simulink model "DK_sim_LFR_diferencial"  (R2020b)
settings: Solver=VariableStepAuto  StartTime=0.0  StopTime=inf  RelTol=1e-3
libraries: vrlib x3
settings Model: Creator=ponyj  LastModifiedBy=ponyj

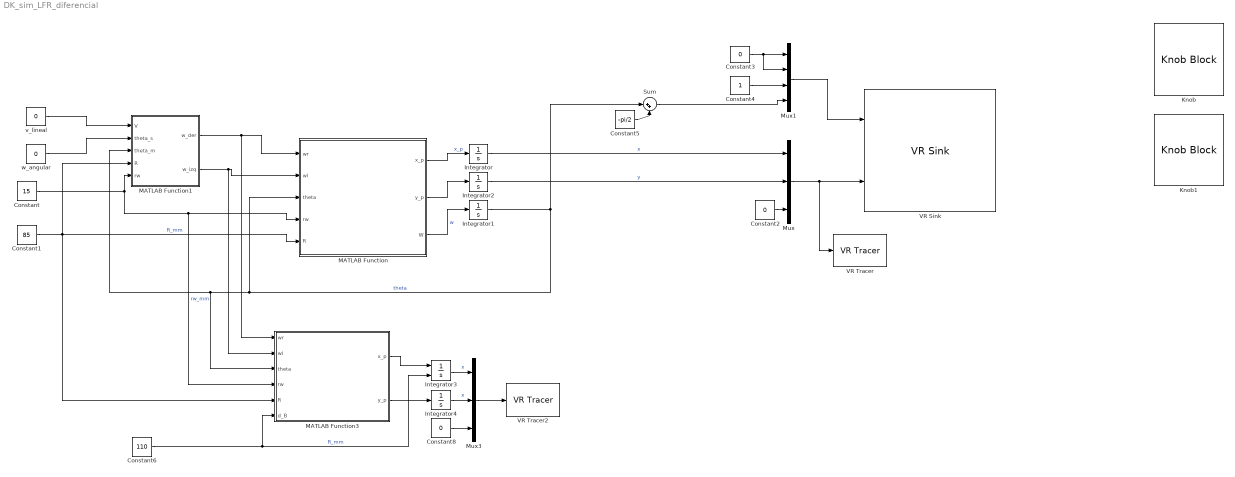
== system DK_sim_LFR_diferencial ==
  Constant : Constant  Value=15
  Constant1 : Constant  Value=85
  Constant2 : Constant  Value=0
  Constant3 : Constant  Value=0
  Constant4 : Constant
  Constant5 : Constant  Value=-pi/2
  Constant6 : Constant  Value=110
  Constant8 : Constant  Value=0
  Integrator{,1..2,4} (4 alike) : Integrator
  Integrator3 : Integrator  InitialConditionSource=external  InitialCondition=1
  Knob : KnobBlock  ScaleMin=-50  ScaleMax=50
  Knob1 : KnobBlock  ScaleMin=-360  ScaleMax=360
  MATLAB Function : MATLAB Function  TreatAsAtomicUnit=on
  MATLAB Function1 : MATLAB Function  TreatAsAtomicUnit=on
  MATLAB Function3 : MATLAB Function  TreatAsAtomicUnit=on
  Mux : Mux  Inputs=3
  Mux1 : Mux
  Mux3 : Mux  Inputs=3
  Sum : Sum  Inputs=|++
  VR Sink : vrlib/VR Sink  InstantiateOnLoad=on  SampleTime=0.1  ViewEnable=on  RemoteChange=off  RemoteView=off  FieldsWritten=LFR_carro.rotation.4.1.1.double#LFR_carro.translation.3.1.1.double  WorldFileName=Mod_Seg_config.wrl  AutoView=off  VideoDimensions=[]  AllowVariableSize=off  FigureProperties="{'Position', 'Name', 'Viewpoint', 'CameraBound', 'CameraDirection', 'CameraPosition', 'CameraUpVector', 'ZoomFactor', 'Antialiasing', 'Headlight', 'Lighting', 'NavPanel', 'Sound', 'StatusBar', 'Stereo3D', 'Stereo3DCameraOffset', 'Stereo3DHIT', 'ToolBar', 'Textures', 'Transparency', 'Triad', 'Wireframe', 'NavZones', 'NavMode', 'NavSpeed', 'CaptureFileFormat', 'CaptureFileName', 'Record2DCompressMethod', 'Record2DCompressQuality', 'Record2D', 'Record2DFileName', 'Record2DFPS'; [1.8000000000000000e+00   8.1399999999999977e+01   7.6640000000000009e+02   6.8280000000000007e+02], '', '_untitled_1', 'on', [0.0000000000000000e+00   0.0000000000000000e+00  -1.0000000000000000e+00], [0.0000000000000000e+00   0.0000000000000000e+00   0.0000000000000000e+00], [0.0000000000000000e+00   1.0000000000000000e+00   0.0000000000000000e+00], [1.0000000000000000e+00], 'on', 'on', 'on', 'halfbar', 'on', 'on', 'off', [1.0000000149011612e-01], [0.0000000000000000e+00], 'on', 'on', 'on', 'none', 'off', 'off', 'fly', 'normal', 'tif', '%f_anim_%n.tif', 'auto', [7.5000000000000000e+01], 'off', '%f_anim_%n.avi', 'auto'}"
  VR Tracer : vrlib/VR Tracer  VrmlFile=Mod_Seg_config.wrl  MarkerName=Tetrahedron  UseLines=on  UseTriads=on  MarkerScale=[1 1 1]  MarkerColorSelection=Selected from color list  MarkerColor=green  rgbval=[1 0 0]  Ts=0.5  ForceViewerOpen=off  ConnectPlane=off  PlaneCoeff=[0 1 0 0]  ConnectPoint=None  PointCoord=[0 0 0]
      settings: SourceProductBaseCode=SL
  VR Tracer2 : vrlib/VR Tracer  VrmlFile=Mod_Seg_config.wrl  MarkerName=Tetrahedron  UseLines=on  UseTriads=on  MarkerScale=[1 1 1]  MarkerColorSelection=Selected from color list  MarkerColor=yellow  rgbval=[1 0 0]  Ts=0.5  ForceViewerOpen=off  ConnectPlane=off  PlaneCoeff=[0 1 0 0]  ConnectPoint=None  PointCoord=[0 0 0]
      settings: SourceProductBaseCode=SL
  v_lineal : Constant  Value=0
  w_angular : Constant  Value=0
  wires:
  Constant/1 -> MATLAB Function3/4(rw), MATLAB Function/4(rw), MATLAB Function1/5(rw)  "rw_mm"
  Constant1/1 -> MATLAB Function3/5(R), MATLAB Function/5(R), MATLAB Function1/4(R)  "R_mm"
  MATLAB Function/1(x_p) -> Integrator/1  "x_p"
  MATLAB Function/3(W) -> Integrator1/1  "w"
  Integrator/1 -> Mux/1  "x"
  Integrator1/1 -> MATLAB Function/3(theta), MATLAB Function3/3(theta), MATLAB Function1/3(theta_m), Sum/1  "theta"
  Mux/1 -> VR Tracer/1, VR Sink/2
  Integrator2/1 -> Mux/2  "y"
  Constant2/1 -> Mux/3
  Mux1/1 -> VR Sink/1
  Constant4/1 -> Mux1/3
  Constant3/1 -> Mux1/2, Mux1/1
  Sum/1 -> Mux1/4
  Constant5/1 -> Sum/2
  v_lineal/1 -> MATLAB Function1/1(V)
  w_angular/1 -> MATLAB Function1/2(theta_s)
  MATLAB Function1/1(w_der) -> MATLAB Function3/1(wr), MATLAB Function/1(wr)
  MATLAB Function/2(y_p) -> Integrator2/1
  Constant6/1 -> Integrator3/2, MATLAB Function3/6(d_B)  "R_mm"
  MATLAB Function1/2(w_izq) -> MATLAB Function/2(wl), MATLAB Function3/2(wl)
  Mux3/1 -> VR Tracer2/1
  Constant8/1 -> Mux3/3
  Integrator4/1 -> Mux3/2  "x"
  Integrator3/1 -> Mux3/1  "x"
  MATLAB Function3/1(x_p) -> Integrator3/1
  MATLAB Function3/2(y_p) -> Integrator4/1

== matlab function DK_sim_LFR_diferencial/MATLAB Function1 ==
  data: V input; w_der output; theta_s input; theta_m input; R input; rw input; w_izq output
function [w_der,w_izq] = fcn(V,theta_s,theta_m, R,rw)

et = theta_s - theta_m*(180/pi);

et = et*(pi/180);

V_der = V + R*et;
V_izq = V - R*et;

w_der = V_der/rw;
w_izq = V_izq/rw;

== matlab function DK_sim_LFR_diferencial/MATLAB Function ==
  data: wr input; wl input; theta input; rw input; R input; x_p output; y_p output; W output
function [x_p,y_p,W] = DK_LFR_Dif(wr,wl,theta,rw,R)

V_l = wl*rw;
V_r = wr*rw;

V = (V_r + V_l)/2;
W = (V_r - V_l)/(2*R);

x_p = V*cos(theta);
y_p = V*sin(theta);

== matlab function DK_sim_LFR_diferencial/MATLAB Function3 ==
  data: wr input; x_p output; wl input; theta input; rw input; R input; d_B input; y_p output
function [x_p,y_p] = DK_SENSORS_LFR_dif(wr,wl,theta,rw,R,d_B)

V_l = wl*rw;
V_r = wr*rw;

V = (V_r + V_l)/2;
W = (V_r - V_l)/(2*R);

x_p = V*cos(theta) -d_B*sin(theta)*W;
y_p = V*sin(theta) +d_B*cos(theta)*W;
